simulink model "costas_loop"  (R2024a)
settings: Solver=FixedStepDiscrete  StartTime=0.0  StopTime=100000.0  RelTol=1e-3
libraries: dspfdesign x2, commdigbbndpm3 x1, commrandsrc3 x1
settings Model: Creator=ISC-03  LastModifiedBy=ISC-03

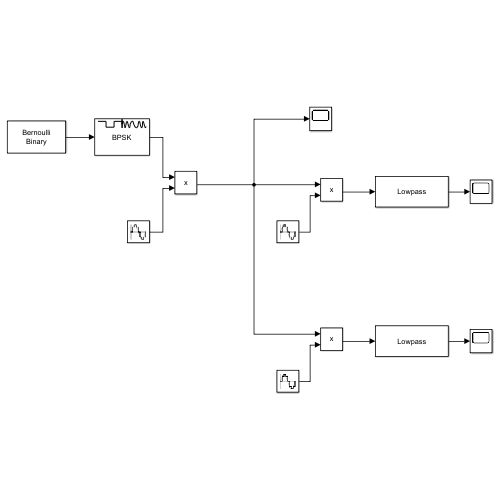
[thumbnail: Simulink's stored preview of the top-level diagram]
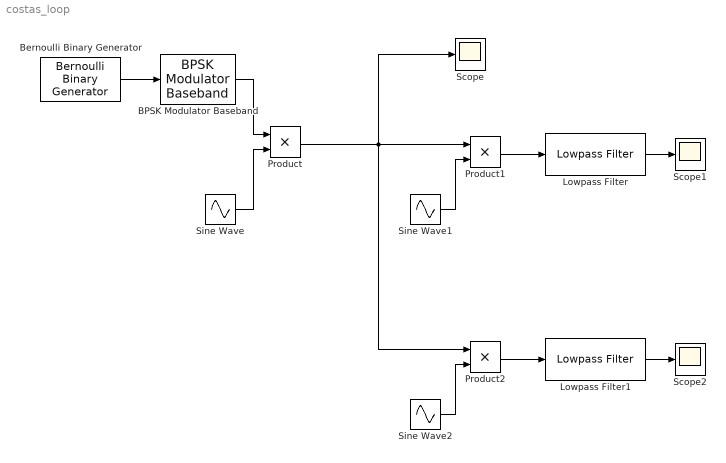
== system costas_loop ==
  BPSK Modulator Baseband : commdigbbndpm3/BPSK Modulator Baseband  Ph=0  outDtype=double  outWordLen=16  outUDDataType=sfix(16)  outFracLenMode=Best precision  outFracLen=15  outDataTypeStr=double  outLastDataTypeStr=double
  Bernoulli Binary Generator : commrandsrc3/Bernoulli Binary Generator  ProbabilityOfZero=0.5  SeedSource=Auto  Seed=0  SampleTime=10000  SamplesPerFrame=1  OutputDataType=boolean  SimulateUsing=Interpreted execution
  Lowpass Filter : dspfdesign/Lowpass Filter  FilterType=FIR  DesignForMinimumOrder=on  FilterOrder=50  PassbandFrequency=0.01  StopbandFrequency=0.1  PassbandRipple=0.1  StopbandAttenuation=80  SampleRateMode=Specify on dialog  SampleRate=1  SimulateUsing=Interpreted execution  roundingMode=Floor  coeffsDataTypeStr=fixdt(1,16)
  Lowpass Filter1 : dspfdesign/Lowpass Filter  FilterType=FIR  DesignForMinimumOrder=on  FilterOrder=50  PassbandFrequency=0.25  StopbandFrequency=0.4  PassbandRipple=0.1  StopbandAttenuation=80  SampleRateMode=Specify on dialog  SampleRate=1  SimulateUsing=Interpreted execution  roundingMode=Floor  coeffsDataTypeStr=fixdt(1,16)
  Product : Product  OutDataTypeStr=double
  Product1 : Product  OutDataTypeStr=double
  Product2 : Product  OutDataTypeStr=double
  Scope : Scope
  Scope1 : Scope
  Scope2 : Scope
  Sine Wave : Sin  Frequency=0.25*pi  Phase=pi/6  SampleTime=1
  Sine Wave1 : Sin  Frequency=0.25*pi  SampleTime=1
  Sine Wave2 : Sin  Frequency=0.25*pi  Phase=pi/2  SampleTime=1
  wires:
  Bernoulli Binary Generator/1 -> BPSK Modulator Baseband/1
  Product/1 -> Product2/1, Product1/1, Scope/1
  BPSK Modulator Baseband/1 -> Product/1
  Sine Wave/1 -> Product/2
  Sine Wave1/1 -> Product1/2
  Sine Wave2/1 -> Product2/2
  Product1/1 -> Lowpass Filter/1
  Lowpass Filter/1 -> Scope1/1
  Product2/1 -> Lowpass Filter1/1
  Lowpass Filter1/1 -> Scope2/1
